simulink model "Q1_sim"  (R2020a)
settings: Solver=ode4  StartTime=0.0  StopTime=20  FixedStep=0.01  RelTol=1e-3
settings Model: Creator=Ali  LastModifiedBy=Ali

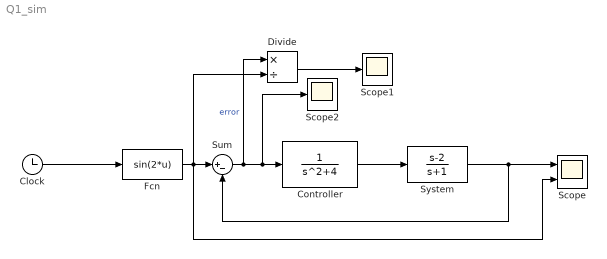
== system Q1_sim ==
  Clock : Clock
  Controller : TransferFcn  Numerator=1  Denominator=[1 0 4]
  Divide : Product  Inputs=*/
  Fcn : Fcn  Expr=sin(2*u)
  Scope : Scope  NumInputPorts=2
  Scope1 : Scope
  Scope2 : Scope
  Sum : Sum  Inputs=|+-
  System : TransferFcn  Numerator=[1 -2]  Denominator=[1 1]
  wires:
  Controller/1 -> System/1
  Clock/1 -> Fcn/1
  Fcn/1 -> Divide/2, Scope/2, Sum/1
  Sum/1 -> Divide/1, Scope2/1, Controller/1  "error"
  System/1 -> Sum/2, Scope/1
  Divide/1 -> Scope1/1
